simulink model "Comparision"  (R2018b)
settings: Solver=VariableStepAuto  StartTime=0.0  StopTime=40  RelTol=1e-3
values from neighbouring files (symbols this model uses):
  N = zeros(3, 7)    [InverseDynamic.m]
  s = (InverseDynamic(jointVelocity,joint ,a) - C)    [ForwardDynamicSolver.m]
undefined symbols (not defined in the file or in its folder): X, Y, Z
libraries: sm_lib x120, nesl_utility x72, simulink x1
(part 1 of 3)
settings Model: Creator=olavoie  LastModifiedBy=olavoie

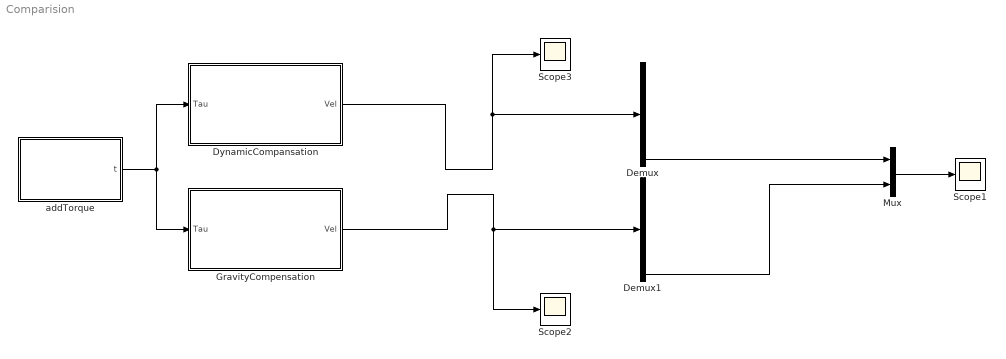
== system Comparision ==
  Demux : Demux  Outputs=7
  Demux1 : Demux  Outputs=7
  DynamicCompansation : Subsystem  TreatAsAtomicUnit=on
  GravityCompensation : Subsystem  TreatAsAtomicUnit=on
  Mux : Mux  Inputs=2
  Scope1 : Scope
  Scope2 : Scope
  Scope3 : Scope
  addTorque : Subsystem  TreatAsAtomicUnit=on
  wires:
  GravityCompensation/1(Vel) -> Demux1/1, Scope2/1
  DynamicCompansation/1(Vel) -> Demux/1, Scope3/1
  addTorque/1(t) -> DynamicCompansation/1(Tau), GravityCompensation/1(Tau)
  Demux1/7 -> Mux/2
  Demux/7 -> Mux/1
  Mux/1 -> Scope1/1

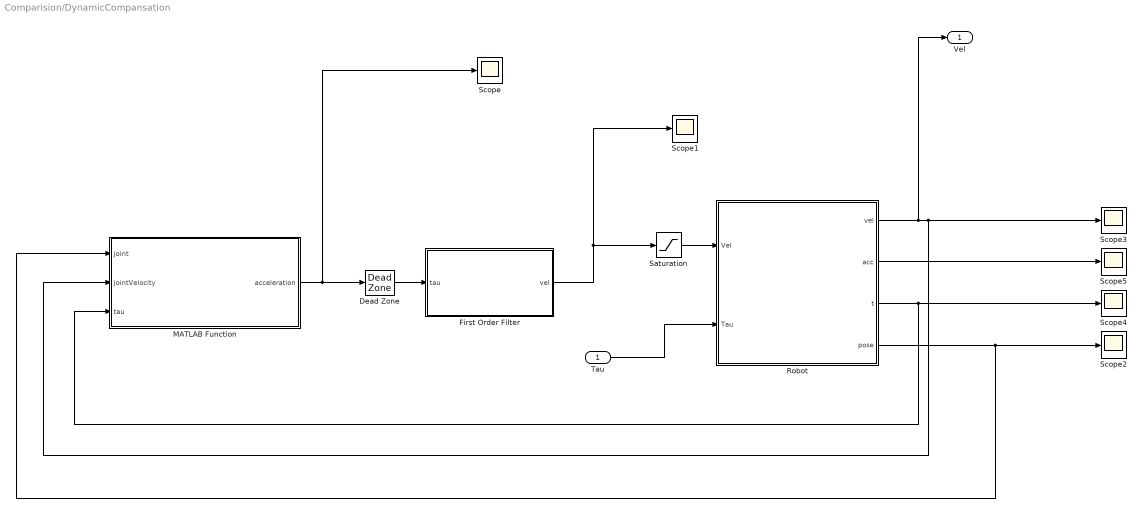
== system Comparision/DynamicCompansation ==
  Tau : Inport
  Dead Zone : DeadZone  LowerValue=-10  UpperValue=10  SaturateOnIntegerOverflow=on
  First Order Filter : Subsystem  TreatAsAtomicUnit=on
  MATLAB Function : MATLAB Function  TreatAsAtomicUnit=on
  Robot : Subsystem  TreatAsAtomicUnit=on
  Saturation : Saturate  UpperLimit=57.3  LowerLimit=-57.3
  Scope{,1..5} (6 alike) : Scope
  Vel : Outport
  wires:
  Robot/3(t) -> MATLAB Function/3(tau), Scope4/1
  Robot/4(pose) -> MATLAB Function/1(joint), Scope2/1
  MATLAB Function/1(acceleration) -> Scope/1, Dead Zone/1
  First Order Filter/1(vel) -> Saturation/1, Scope1/1
  Robot/2(acc) -> Scope5/1
  Robot/1(vel) -> Vel/1, MATLAB Function/2(jointVelocity), Scope3/1
  Dead Zone/1 -> First Order Filter/1(tau)
  Tau/1 -> Robot/2(Tau)
  Saturation/1 -> Robot/1(Vel)

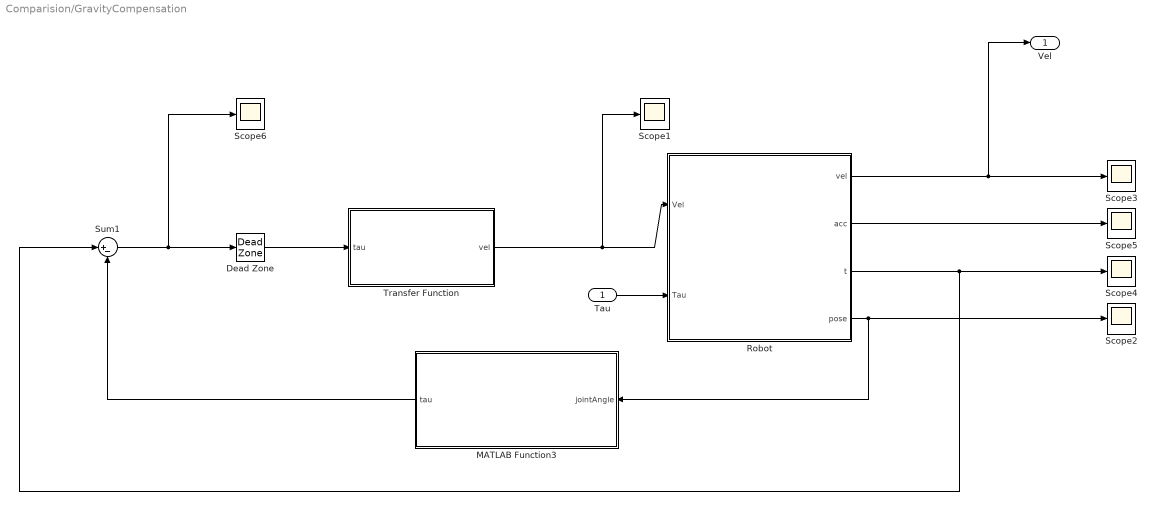
== system Comparision/GravityCompensation ==
  Tau : Inport
  Dead Zone : DeadZone  LowerValue=-10  UpperValue=10  SaturateOnIntegerOverflow=on
  MATLAB Function3 : MATLAB Function  TreatAsAtomicUnit=on
  Robot : Subsystem  TreatAsAtomicUnit=on
  Scope{1..6} (6 alike) : Scope
  Sum1 : Sum  Inputs=|+-
  Transfer Function : Subsystem  TreatAsAtomicUnit=on
  Vel : Outport
  wires:
  Robot/4(pose) -> Scope2/1, MATLAB Function3/1(jointAngle)
  Robot/2(acc) -> Scope5/1
  Robot/3(t) -> Scope4/1, Sum1/1
  Transfer Function/1(vel) -> Scope1/1, Robot/1(Vel)
  MATLAB Function3/1(tau) -> Sum1/2
  Dead Zone/1 -> Transfer Function/1(tau)
  Sum1/1 -> Scope6/1, Dead Zone/1
  Robot/1(vel) -> Vel/1, Scope3/1
  Tau/1 -> Robot/2(Tau)

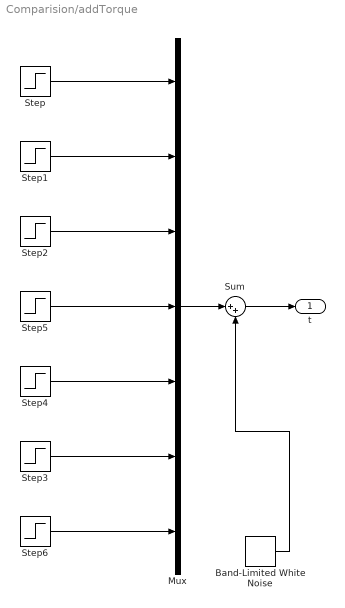
== system Comparision/addTorque ==
  Band-Limited White Noise : simulink/Sources/Band-Limited White Noise  Cov=[0.5]  Ts=0.001  seed=[23341]
  Mux : Mux  Inputs=7
  Step : Step  Time=0  After=100  SampleTime=0
  Step{1..6} (6 alike) : Step  Time=0  After=0  SampleTime=0
  Sum : Sum  Inputs=|++
  t : Outport
  wires:
  Step/1 -> Mux/1
  Step6/1 -> Mux/7
  Step3/1 -> Mux/6
  Step4/1 -> Mux/5
  Step5/1 -> Mux/4
  Step2/1 -> Mux/3
  Step1/1 -> Mux/2
  Mux/1 -> Sum/1
  Sum/1 -> t/1
  Band-Limited White Noise/1 -> Sum/2

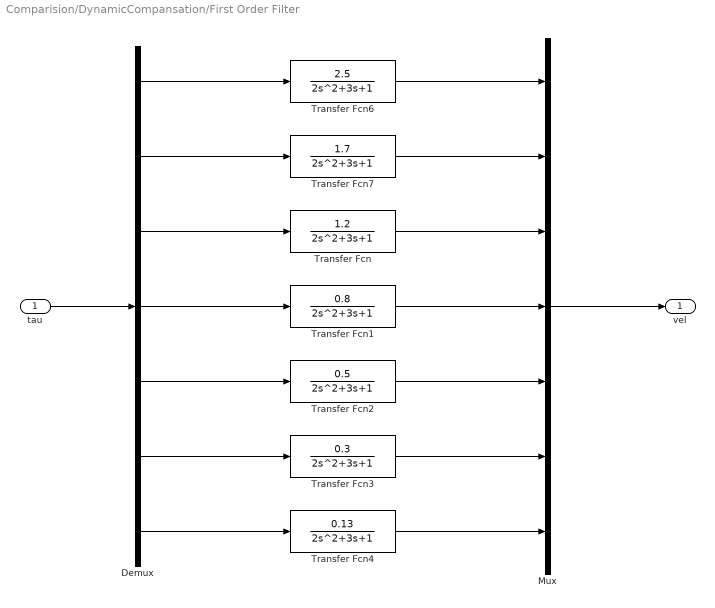
== system Comparision/DynamicCompansation/First Order Filter ==
  tau : Inport
  Demux : Demux  Outputs=7
  Mux : Mux  Inputs=7
  Transfer Fcn : TransferFcn  Numerator=[1.2]  Denominator=[2 3 1]
  Transfer Fcn1 : TransferFcn  Numerator=[0.8]  Denominator=[2 3 1]
  Transfer Fcn2 : TransferFcn  Numerator=[0.5]  Denominator=[2 3 1]
  Transfer Fcn3 : TransferFcn  Numerator=[0.3]  Denominator=[2 3 1]
  Transfer Fcn4 : TransferFcn  Numerator=[0.13]  Denominator=[2 3 1]
  Transfer Fcn6 : TransferFcn  Numerator=[2.5]  Denominator=[2 3 1]
  Transfer Fcn7 : TransferFcn  Numerator=[1.7]  Denominator=[2 3 1]
  vel : Outport
  wires:
  Transfer Fcn2/1 -> Mux/5
  Demux/7 -> Transfer Fcn4/1
  Transfer Fcn1/1 -> Mux/4
  Transfer Fcn4/1 -> Mux/7
  Transfer Fcn/1 -> Mux/3
  Demux/3 -> Transfer Fcn/1
  Demux/5 -> Transfer Fcn2/1
  Transfer Fcn7/1 -> Mux/2
  Transfer Fcn3/1 -> Mux/6
  Mux/1 -> vel/1
  Demux/4 -> Transfer Fcn1/1
  tau/1 -> Demux/1
  Demux/6 -> Transfer Fcn3/1
  Transfer Fcn6/1 -> Mux/1
  Demux/2 -> Transfer Fcn7/1
  Demux/1 -> Transfer Fcn6/1

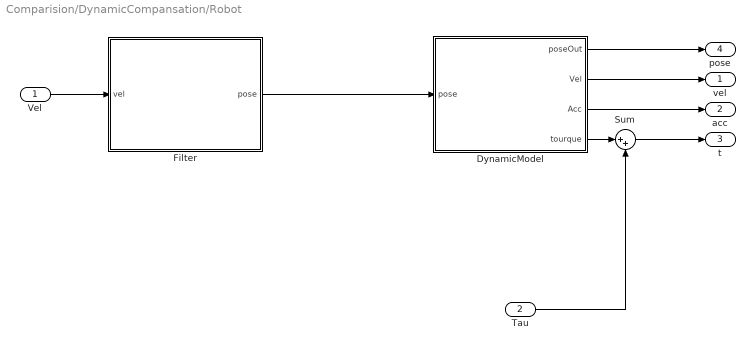
== system Comparision/DynamicCompansation/Robot ==
  Vel : Inport
  Tau : Inport  Port=2
  DynamicModel : Subsystem  TreatAsAtomicUnit=on
  Filter : Subsystem  TreatAsAtomicUnit=on
  Sum : Sum  Inputs=|++
  vel : Outport
  acc : Outport  Port=2
  t : Outport  Port=3
  pose : Outport  Port=4
  wires:
  Vel/1 -> Filter/1(vel)
  Filter/1(pose) -> DynamicModel/1(pose)
  DynamicModel/1(poseOut) -> pose/1
  DynamicModel/2(Vel) -> vel/1
  DynamicModel/3(Acc) -> acc/1
  DynamicModel/4(tourque) -> Sum/1
  Sum/1 -> t/1
  Tau/1 -> Sum/2

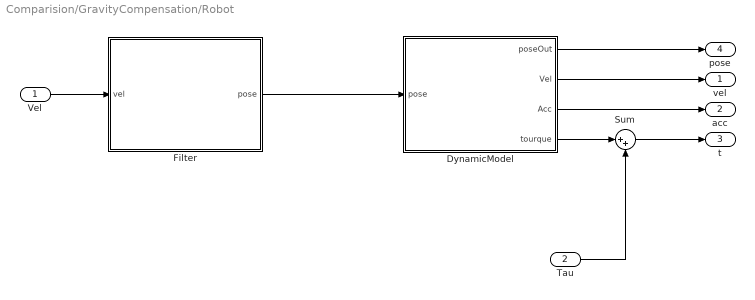
== system Comparision/GravityCompensation/Robot ==
  Vel : Inport
  Tau : Inport  Port=2
  DynamicModel : Subsystem  TreatAsAtomicUnit=on
  Filter : Subsystem  TreatAsAtomicUnit=on
  Sum : Sum  Inputs=|++
  vel : Outport
  acc : Outport  Port=2
  t : Outport  Port=3
  pose : Outport  Port=4
  wires:
  Vel/1 -> Filter/1(vel)
  Filter/1(pose) -> DynamicModel/1(pose)
  DynamicModel/1(poseOut) -> pose/1
  DynamicModel/2(Vel) -> vel/1
  DynamicModel/3(Acc) -> acc/1
  DynamicModel/4(tourque) -> Sum/1
  Sum/1 -> t/1
  Tau/1 -> Sum/2

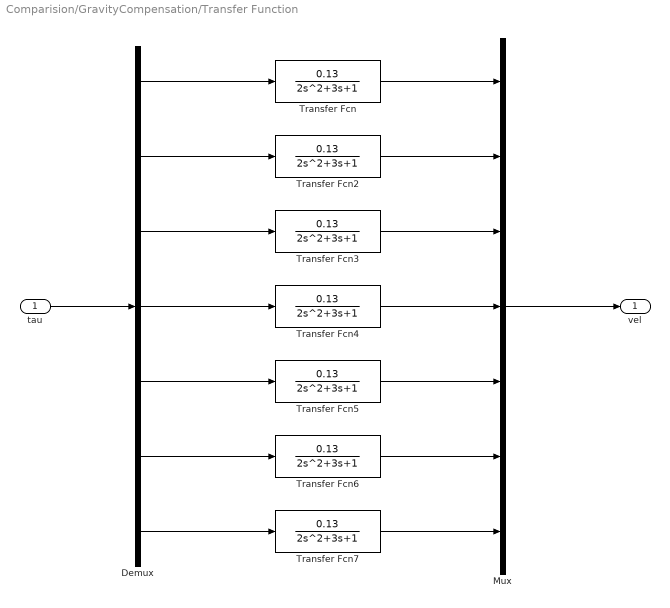
== system Comparision/GravityCompensation/Transfer Function ==
  tau : Inport
  Demux : Demux  Outputs=7
  Mux : Mux  Inputs=7
  Transfer Fcn{,2..7} (7 alike) : TransferFcn  Numerator=[0.13]  Denominator=[2 3 1]
  vel : Outport
  wires:
  Demux/1 -> Transfer Fcn/1
  Demux/2 -> Transfer Fcn2/1
  Demux/3 -> Transfer Fcn3/1
  Demux/4 -> Transfer Fcn4/1
  Demux/5 -> Transfer Fcn5/1
  Demux/6 -> Transfer Fcn6/1
  Demux/7 -> Transfer Fcn7/1
  Transfer Fcn/1 -> Mux/1
  Transfer Fcn2/1 -> Mux/2
  Transfer Fcn3/1 -> Mux/3
  Transfer Fcn4/1 -> Mux/4
  Transfer Fcn5/1 -> Mux/5
  Transfer Fcn6/1 -> Mux/6
  Transfer Fcn7/1 -> Mux/7
  tau/1 -> Demux/1
  Mux/1 -> vel/1

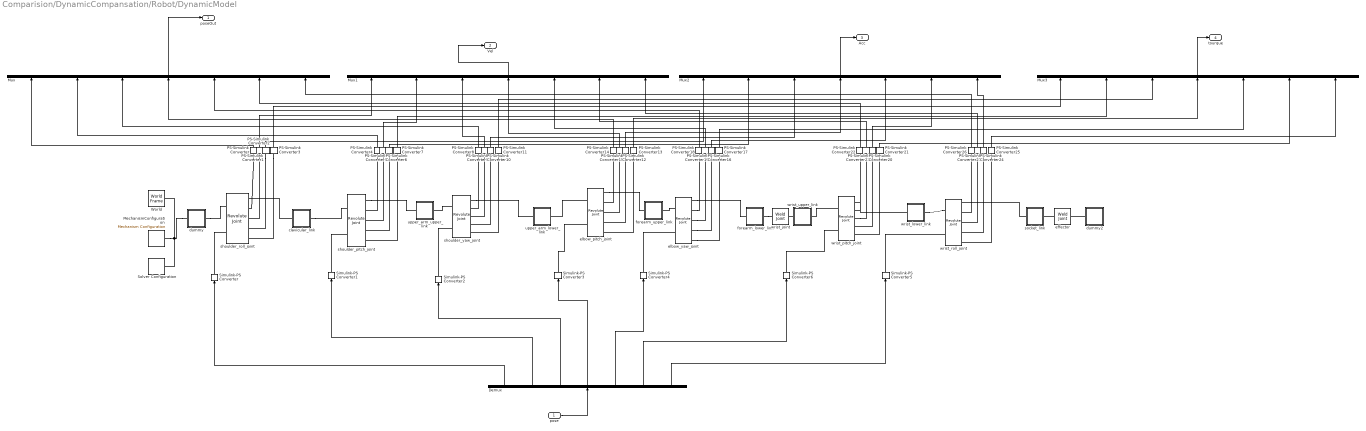
== system Comparision/DynamicCompansation/Robot/DynamicModel ==
  pose : Inport
  Demux : Demux  Outputs=7
  MechanismConfiguration : sm_lib/Utilities/Mechanism Configuration  UniformGravity=Constant  GravityVector=[0 0 -9.81]  GravityUnits=m/s^2  LinearizationDelta=0.001
  Mux{,1..3} (4 alike) : Mux  Inputs=7
  PS-Simulink Converter{,1..27} (28 alike) : nesl_utility/PS-Simulink Converter  PhysicalDomain=network_engine_domain  SubClassName=ps_output  LeftPortType=input  RightPortType=output  PseudoPeriodic=off  Frequencies=[]  Unit=1  AffineConversion=off
  Simulink-PS Converter{,1..6} (7 alike) : nesl_utility/Simulink-PS Converter  PhysicalDomain=network_engine_domain  SubClassName=ps_input  LeftPortType=input  RightPortType=output  PseudoPeriodic=off  Frequencies=[]  NoiseDistribution=none  NoiseParameters=[]  Unit=rad  AffineConversion=off  FilteringAndDerivatives=filter  SimscapeFilterOrder=2  InputFilterTimeConstant=0.001  UdotUserProvided=0
  Solver Configuration : nesl_utility/Solver Configuration  PhysicalDomain=network_engine_domain  SubClassName=solver  LeftPortType=input  RightPortType=generic  Tones=[]  Harmonics=[]  SimulateNoise=off  Profile=off  UseLocalSampling=off  EnableSwitchedLinearOptims=on  FrequencyDomain=off  UseCCode=off  RelTol=0.001  AbsTol=1e-06  MinStep=1e-09  ToWorkspace=off  RevertToSquareIcSolve=off  NumHomotopyIterations=100  PhasorMode=off  PhasorModeNumHarmonics=1  DoDC=off  ResidualTolerance=1e-09  UseLocalSolver=off  LocalSolverChoice=NE_BACKWARD_EULER_ADVANCER  LocalSolverSampleTime=0.001  DoFixedCost=off  MaxNonlinIter=3  MaxModeIter=2  LinearAlgebra=auto  EquationFormulation=NE_TIME_EF  DelaysMemoryBudget=1024  AutomaticFiltering=on  FilteringTimeConstant=0.001  PartitionStorageMethod=AS_NEEDED  PartitionMemoryBudget=1024
  World : sm_lib/Frames and Transforms/World Frame
  clavicular_link : Subsystem
  dummy : Subsystem
  dummy2 : Subsystem
  effector : sm_lib/Joints/Weld Joint  SenseConstraintForce=off  SenseConstraintForceX=off  SenseConstraintForceY=off  SenseConstraintForceZ=off  SenseConstraintTorque=off  SenseConstraintTorqueX=off  SenseConstraintTorqueY=off  SenseConstraintTorqueZ=off  SenseTotalForce=off  SenseTotalForceX=off  SenseTotalForceY=off  SenseTotalForceZ=off  SenseTotalTorque=off  SenseTotalTorqueX=off  SenseTotalTorqueY=off  SenseTotalTorqueZ=off  CompositeWrenchDir=FollowerOnBase  CompositeWrenchFrame=BaseFrame
  elbow_pitch_joint : sm_lib/Joints/Revolute Joint  SenseConstraintForce=off  SenseConstraintForceX=off  SenseConstraintForceY=off  SenseConstraintForceZ=off  SenseConstraintTorque=off  SenseConstraintTorqueX=off  SenseConstraintTorqueY=off  SenseConstraintTorqueZ=off  SenseTotalForce=off  SenseTotalForceX=off  SenseTotalForceY=off  SenseTotalForceZ=off  SenseTotalTorque=off  SenseTotalTorqueX=off  SenseTotalTorqueY=off  SenseTotalTorqueZ=off  CompositeWrenchDir=FollowerOnBase  CompositeWrenchFrame=BaseFrame  EquilibriumPosition=0  EquilibriumPositionUnits=deg  SpringStiffness=0  SpringStiffnessUnits=N*m/deg  DampingCoefficient=0.1  DampingCoefficientUnits=m^2*kg/s/rad  TorqueActuationMode=ComputedTorque  MotionActuationMode=InputMotion  SensePosition=on  SenseVelocity=on  SenseAcceleration=on  SenseTorqueForce=on  PositionTargetSpecify=off  PositionTargetPriority=High  PositionTargetValue=0  PositionTargetValueUnits=deg  VelocityTargetSpecify=off  VelocityTargetPriority=High  VelocityTargetValue=0  VelocityTargetValueUnits=deg/s
  elbow_yaw_joint : sm_lib/Joints/Revolute Joint  SenseConstraintForce=off  SenseConstraintForceX=off  SenseConstraintForceY=off  SenseConstraintForceZ=off  SenseConstraintTorque=off  SenseConstraintTorqueX=off  SenseConstraintTorqueY=off  SenseConstraintTorqueZ=off  SenseTotalForce=off  SenseTotalForceX=off  SenseTotalForceY=off  SenseTotalForceZ=off  SenseTotalTorque=off  SenseTotalTorqueX=off  SenseTotalTorqueY=off  SenseTotalTorqueZ=off  CompositeWrenchDir=FollowerOnBase  CompositeWrenchFrame=BaseFrame  EquilibriumPosition=0  EquilibriumPositionUnits=deg  SpringStiffness=0  SpringStiffnessUnits=N*m/deg  DampingCoefficient=0.1  DampingCoefficientUnits=m^2*kg/s/rad  TorqueActuationMode=ComputedTorque  MotionActuationMode=InputMotion  SensePosition=on  SenseVelocity=on  SenseAcceleration=on  SenseTorqueForce=on  PositionTargetSpecify=off  PositionTargetPriority=High  PositionTargetValue=0  PositionTargetValueUnits=deg  VelocityTargetSpecify=off  VelocityTargetPriority=High  VelocityTargetValue=0  VelocityTargetValueUnits=deg/s
  forearm_lower_link : Subsystem
  forearm_upper_link : Subsystem
  shoulder_pitch_joint : sm_lib/Joints/Revolute Joint  SenseConstraintForce=off  SenseConstraintForceX=off  SenseConstraintForceY=off  SenseConstraintForceZ=off  SenseConstraintTorque=off  SenseConstraintTorqueX=off  SenseConstraintTorqueY=off  SenseConstraintTorqueZ=off  SenseTotalForce=off  SenseTotalForceX=off  SenseTotalForceY=off  SenseTotalForceZ=off  SenseTotalTorque=off  SenseTotalTorqueX=off  SenseTotalTorqueY=off  SenseTotalTorqueZ=off  CompositeWrenchDir=FollowerOnBase  CompositeWrenchFrame=BaseFrame  EquilibriumPosition=0  EquilibriumPositionUnits=deg  SpringStiffness=0  SpringStiffnessUnits=N*m/deg  DampingCoefficient=0.1  DampingCoefficientUnits=m^2*kg/s/rad  TorqueActuationMode=ComputedTorque  MotionActuationMode=InputMotion  SensePosition=on  SenseVelocity=on  SenseAcceleration=on  SenseTorqueForce=on  PositionTargetSpecify=off  PositionTargetPriority=High  PositionTargetValue=0  PositionTargetValueUnits=deg  VelocityTargetSpecify=off  VelocityTargetPriority=High  VelocityTargetValue=0  VelocityTargetValueUnits=deg/s
  shoulder_roll_joint : sm_lib/Joints/Revolute Joint  SenseConstraintForce=off  SenseConstraintForceX=off  SenseConstraintForceY=off  SenseConstraintForceZ=off  SenseConstraintTorque=off  SenseConstraintTorqueX=off  SenseConstraintTorqueY=off  SenseConstraintTorqueZ=off  SenseTotalForce=off  SenseTotalForceX=off  SenseTotalForceY=off  SenseTotalForceZ=off  SenseTotalTorque=off  SenseTotalTorqueX=off  SenseTotalTorqueY=off  SenseTotalTorqueZ=off  CompositeWrenchDir=FollowerOnBase  CompositeWrenchFrame=FollowerFrame  EquilibriumPosition=0  EquilibriumPositionUnits=deg  SpringStiffness=0  SpringStiffnessUnits=N*m/deg  DampingCoefficient=0.1  DampingCoefficientUnits=m^2*kg/s/rad  TorqueActuationMode=ComputedTorque  MotionActuationMode=InputMotion  SensePosition=on  SenseVelocity=on  SenseAcceleration=on  SenseTorqueForce=on  PositionTargetSpecify=on  PositionTargetPriority=High  PositionTargetValue=0  PositionTargetValueUnits=deg  VelocityTargetSpecify=on  VelocityTargetPriority=High  VelocityTargetValue=0  VelocityTargetValueUnits=deg/s
  shoulder_yaw_joint : sm_lib/Joints/Revolute Joint  SenseConstraintForce=off  SenseConstraintForceX=off  SenseConstraintForceY=off  SenseConstraintForceZ=off  SenseConstraintTorque=off  SenseConstraintTorqueX=off  SenseConstraintTorqueY=off  SenseConstraintTorqueZ=off  SenseTotalForce=off  SenseTotalForceX=off  SenseTotalForceY=off  SenseTotalForceZ=off  SenseTotalTorque=off  SenseTotalTorqueX=off  SenseTotalTorqueY=off  SenseTotalTorqueZ=off  CompositeWrenchDir=FollowerOnBase  CompositeWrenchFrame=FollowerFrame  EquilibriumPosition=0  EquilibriumPositionUnits=deg  SpringStiffness=0  SpringStiffnessUnits=N*m/deg  DampingCoefficient=0.1  DampingCoefficientUnits=m^2*kg/s/rad  TorqueActuationMode=ComputedTorque  MotionActuationMode=InputMotion  SensePosition=on  SenseVelocity=on  SenseAcceleration=on  SenseTorqueForce=on  PositionTargetSpecify=off  PositionTargetPriority=High  PositionTargetValue=0  PositionTargetValueUnits=deg  VelocityTargetSpecify=off  VelocityTargetPriority=High  VelocityTargetValue=0  VelocityTargetValueUnits=deg/s
  socket_link : Subsystem
  upper_arm_lower_link : Subsystem
  upper_arm_upper_link : Subsystem
  wrist_joint : sm_lib/Joints/Weld Joint  SenseConstraintForce=off  SenseConstraintForceX=off  SenseConstraintForceY=off  SenseConstraintForceZ=off  SenseConstraintTorque=off  SenseConstraintTorqueX=off  SenseConstraintTorqueY=off  SenseConstraintTorqueZ=off  SenseTotalForce=off  SenseTotalForceX=off  SenseTotalForceY=off  SenseTotalForceZ=off  SenseTotalTorque=off  SenseTotalTorqueX=off  SenseTotalTorqueY=off  SenseTotalTorqueZ=off  CompositeWrenchDir=FollowerOnBase  CompositeWrenchFrame=BaseFrame
  wrist_lower_link : Subsystem
  wrist_pitch_joint : sm_lib/Joints/Revolute Joint  SenseConstraintForce=off  SenseConstraintForceX=off  SenseConstraintForceY=off  SenseConstraintForceZ=off  SenseConstraintTorque=off  SenseConstraintTorqueX=off  SenseConstraintTorqueY=off  SenseConstraintTorqueZ=off  SenseTotalForce=off  SenseTotalForceX=off  SenseTotalForceY=off  SenseTotalForceZ=off  SenseTotalTorque=off  SenseTotalTorqueX=off  SenseTotalTorqueY=off  SenseTotalTorqueZ=off  CompositeWrenchDir=FollowerOnBase  CompositeWrenchFrame=BaseFrame  EquilibriumPosition=0  EquilibriumPositionUnits=deg  SpringStiffness=0  SpringStiffnessUnits=N*m/deg  DampingCoefficient=0.1  DampingCoefficientUnits=m^2*kg/s/rad  TorqueActuationMode=ComputedTorque  MotionActuationMode=InputMotion  SensePosition=on  SenseVelocity=on  SenseAcceleration=on  SenseTorqueForce=on  PositionTargetSpecify=off  PositionTargetPriority=High  PositionTargetValue=0  PositionTargetValueUnits=deg  VelocityTargetSpecify=off  VelocityTargetPriority=High  VelocityTargetValue=0  VelocityTargetValueUnits=deg/s
  wrist_roll_joint : sm_lib/Joints/Revolute Joint  SenseConstraintForce=off  SenseConstraintForceX=off  SenseConstraintForceY=off  SenseConstraintForceZ=off  SenseConstraintTorque=off  SenseConstraintTorqueX=off  SenseConstraintTorqueY=off  SenseConstraintTorqueZ=off  SenseTotalForce=off  SenseTotalForceX=off  SenseTotalForceY=off  SenseTotalForceZ=off  SenseTotalTorque=off  SenseTotalTorqueX=off  SenseTotalTorqueY=off  SenseTotalTorqueZ=off  CompositeWrenchDir=FollowerOnBase  CompositeWrenchFrame=BaseFrame  EquilibriumPosition=0  EquilibriumPositionUnits=deg  SpringStiffness=0  SpringStiffnessUnits=N*m/deg  DampingCoefficient=0.1  DampingCoefficientUnits=m^2*kg/s/rad  TorqueActuationMode=ComputedTorque  MotionActuationMode=InputMotion  SensePosition=on  SenseVelocity=on  SenseAcceleration=on  SenseTorqueForce=on  PositionTargetSpecify=off  PositionTargetPriority=High  PositionTargetValue=0  PositionTargetValueUnits=deg  VelocityTargetSpecify=off  VelocityTargetPriority=High  VelocityTargetValue=0  VelocityTargetValueUnits=deg/s
  wrist_upper_link : Subsystem
  poseOut : Outport
  Vel : Outport  Port=2
  Acc : Outport  Port=3
  tourque : Outport  Port=4
  wires:
  PS-Simulink Converter23/1 -> Mux1/6
  PS-Simulink Converter25/1 -> Mux3/7
  PS-Simulink Converter12/1 -> Mux2/4
  PS-Simulink Converter16/1 -> Mux2/5
  Mux1/1 -> Vel/1
  PS-Simulink Converter19/1 -> Mux1/5
  PS-Simulink Converter27/1 -> Mux1/7
  Demux/7 -> Simulink-PS Converter5/1
  PS-Simulink Converter/1 -> Mux/1
  PS-Simulink Converter20/1 -> Mux2/6
  Mux3/1 -> tourque/1
  Demux/1 -> Simulink-PS Converter/1
  PS-Simulink Converter22/1 -> Mux/6
  Mux2/1 -> Acc/1
  PS-Simulink Converter7/1 -> Mux3/2
  PS-Simulink Converter26/1 -> Mux/7
  PS-Simulink Converter10/1 -> Mux2/3
  Demux/6 -> Simulink-PS Converter6/1
  PS-Simulink Converter18/1 -> Mux/5
  PS-Simulink Converter24/1 -> Mux2/7
  PS-Simulink Converter14/1 -> Mux/4
  PS-Simulink Converter5/1 -> Mux1/2
  PS-Simulink Converter17/1 -> Mux3/5
  PS-Simulink Converter21/1 -> Mux3/6
  Demux/5 -> Simulink-PS Converter4/1
  PS-Simulink Converter2/1 -> Mux2/1
  PS-Simulink Converter8/1 -> Mux/3
  PS-Simulink Converter13/1 -> Mux3/4
  PS-Simulink Converter11/1 -> Mux3/3
  Mux/1 -> poseOut/1
  PS-Simulink Converter9/1 -> Mux1/3
  PS-Simulink Converter15/1 -> Mux1/4
  PS-Simulink Converter3/1 -> Mux3/1
  PS-Simulink Converter1/1 -> Mux1/1
  PS-Simulink Converter6/1 -> Mux2/2
  Demux/2 -> Simulink-PS Converter1/1
  PS-Simulink Converter4/1 -> Mux/2
  Demux/3 -> Simulink-PS Converter2/1
  pose/1 -> Demux/1
  Demux/4 -> Simulink-PS Converter3/1
  connections:
  dummy/LConn1 -- MechanismConfiguration/RConn1 -- Solver Configuration/RConn1 -- World/RConn1
  elbow_yaw_joint/RConn1 -- forearm_lower_link/LConn1
  PS-Simulink Converter3/LConn1 -- shoulder_roll_joint/RConn5
  elbow_yaw_joint/RConn5 -- PS-Simulink Converter17/LConn1
  PS-Simulink Converter6/LConn1 -- shoulder_pitch_joint/RConn4
  wrist_lower_link/LConn1 -- wrist_pitch_joint/RConn1
  PS-Simulink Converter14/LConn1 -- elbow_pitch_joint/RConn2
  PS-Simulink Converter5/LConn1 -- shoulder_pitch_joint/RConn3
  shoulder_yaw_joint/LConn2 -- Simulink-PS Converter2/RConn1
  clavicular_link/LConn1 -- shoulder_roll_joint/RConn1
  PS-Simulink Converter12/LConn1 -- elbow_pitch_joint/RConn4
  wrist_pitch_joint/RConn2 -- PS-Simulink Converter22/LConn1
  PS-Simulink Converter24/LConn1 -- wrist_roll_joint/RConn4
  Simulink-PS Converter6/RConn1 -- wrist_pitch_joint/LConn2
  PS-Simulink Converter4/LConn1 -- shoulder_pitch_joint/RConn2
  PS-Simulink Converter21/LConn1 -- wrist_pitch_joint/RConn5
  PS-Simulink Converter13/LConn1 -- elbow_pitch_joint/RConn5
  socket_link/LConn1 -- wrist_roll_joint/RConn1
  PS-Simulink Converter/LConn1 -- shoulder_roll_joint/RConn2
  PS-Simulink Converter2/LConn1 -- shoulder_roll_joint/RConn4
  elbow_yaw_joint/RConn2 -- PS-Simulink Converter18/LConn1
  PS-Simulink Converter1/LConn1 -- shoulder_roll_joint/RConn3
  PS-Simulink Converter25/LConn1 -- wrist_roll_joint/RConn5
  shoulder_pitch_joint/RConn1 -- upper_arm_upper_link/LConn1
  PS-Simulink Converter10/LConn1 -- shoulder_yaw_joint/RConn4
  PS-Simulink Converter7/LConn1 -- shoulder_pitch_joint/RConn5
  elbow_pitch_joint/LConn2 -- Simulink-PS Converter3/RConn1
  PS-Simulink Converter27/LConn1 -- wrist_roll_joint/RConn3
  dummy2/LConn1 -- effector/RConn1
  elbow_yaw_joint/RConn3 -- PS-Simulink Converter19/LConn1
  shoulder_yaw_joint/RConn1 -- upper_arm_lower_link/LConn1
  PS-Simulink Converter11/LConn1 -- shoulder_yaw_joint/RConn5
  wrist_lower_link/RConn1 -- wrist_roll_joint/LConn1
  PS-Simulink Converter26/LConn1 -- wrist_roll_joint/RConn2
  shoulder_yaw_joint/LConn1 -- upper_arm_upper_link/RConn1
  wrist_joint/RConn1 -- wrist_upper_link/LConn1
  PS-Simulink Converter20/LConn1 -- wrist_pitch_joint/RConn4
  elbow_yaw_joint/LConn2 -- Simulink-PS Converter4/RConn1
  forearm_lower_link/RConn1 -- wrist_joint/LConn1
  effector/LConn1 -- socket_link/RConn1
  Simulink-PS Converter1/RConn1 -- shoulder_pitch_joint/LConn2
  elbow_pitch_joint/RConn1 -- forearm_upper_link/LConn1
  elbow_pitch_joint/LConn1 -- upper_arm_lower_link/RConn1
  dummy/RConn1 -- shoulder_roll_joint/LConn1
  PS-Simulink Converter15/LConn1 -- elbow_pitch_joint/RConn3
  wrist_pitch_joint/RConn3 -- PS-Simulink Converter23/LConn1
  elbow_yaw_joint/RConn4 -- PS-Simulink Converter16/LConn1
  clavicular_link/RConn1 -- shoulder_pitch_joint/LConn1
  Simulink-PS Converter5/RConn1 -- wrist_roll_joint/LConn2
  wrist_pitch_joint/LConn1 -- wrist_upper_link/RConn1
  PS-Simulink Converter8/LConn1 -- shoulder_yaw_joint/RConn2
  PS-Simulink Converter9/LConn1 -- shoulder_yaw_joint/RConn3
  elbow_yaw_joint/LConn1 -- forearm_upper_link/RConn1
  Simulink-PS Converter/RConn1 -- shoulder_roll_joint/LConn2

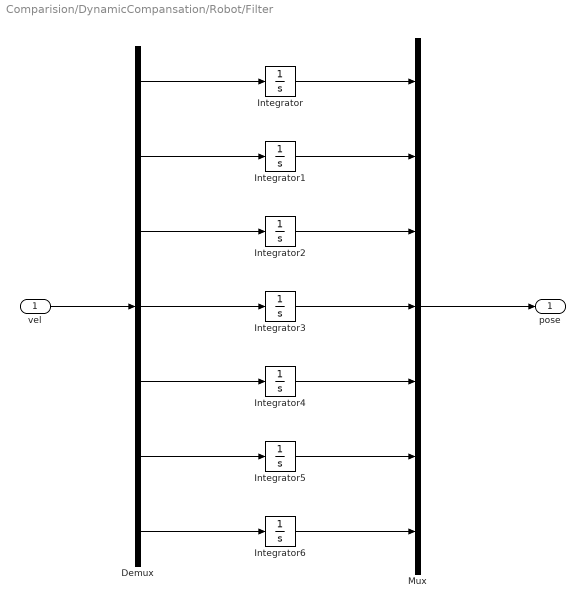
== system Comparision/DynamicCompansation/Robot/Filter ==
  vel : Inport
  Demux : Demux  Outputs=7
  Integrator{,1..6} (7 alike) : Integrator
  Mux : Mux  Inputs=7
  pose : Outport
  wires:
  Mux/1 -> pose/1
  Demux/1 -> Integrator/1
  Integrator/1 -> Mux/1
  Demux/7 -> Integrator6/1
  Integrator6/1 -> Mux/7
  Demux/6 -> Integrator5/1
  Integrator5/1 -> Mux/6
  Demux/5 -> Integrator4/1
  Integrator4/1 -> Mux/5
  Demux/4 -> Integrator3/1
  Integrator3/1 -> Mux/4
  Demux/3 -> Integrator2/1
  Integrator2/1 -> Mux/3
  Demux/2 -> Integrator1/1
  Integrator1/1 -> Mux/2
  vel/1 -> Demux/1

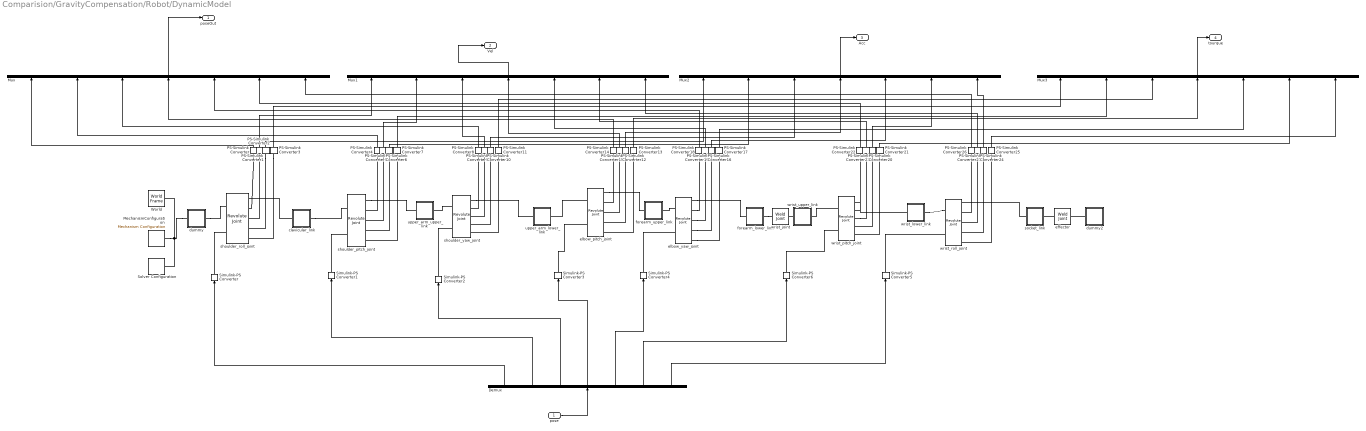
== system Comparision/GravityCompensation/Robot/DynamicModel ==
  pose : Inport
  Demux : Demux  Outputs=7
  MechanismConfiguration : sm_lib/Utilities/Mechanism Configuration  UniformGravity=Constant  GravityVector=[0 0 9.81]  GravityUnits=m/s^2  LinearizationDelta=0.001
  Mux{,1..3} (4 alike) : Mux  Inputs=7
  PS-Simulink Converter{,1..27} (28 alike) : nesl_utility/PS-Simulink Converter  PhysicalDomain=network_engine_domain  SubClassName=ps_output  LeftPortType=input  RightPortType=output  PseudoPeriodic=off  Frequencies=[]  Unit=1  AffineConversion=off
  Simulink-PS Converter{,1..6} (7 alike) : nesl_utility/Simulink-PS Converter  PhysicalDomain=network_engine_domain  SubClassName=ps_input  LeftPortType=input  RightPortType=output  PseudoPeriodic=off  Frequencies=[]  NoiseDistribution=none  NoiseParameters=[]  Unit=rad  AffineConversion=off  FilteringAndDerivatives=filter  SimscapeFilterOrder=2  InputFilterTimeConstant=0.001  UdotUserProvided=0
  Solver Configuration : nesl_utility/Solver Configuration  PhysicalDomain=network_engine_domain  SubClassName=solver  LeftPortType=input  RightPortType=generic  Tones=[]  Harmonics=[]  SimulateNoise=off  Profile=off  UseLocalSampling=off  EnableSwitchedLinearOptims=on  FrequencyDomain=off  UseCCode=off  RelTol=0.001  AbsTol=1e-06  MinStep=1e-09  ToWorkspace=off  RevertToSquareIcSolve=off  NumHomotopyIterations=100  PhasorMode=off  PhasorModeNumHarmonics=1  DoDC=off  ResidualTolerance=1e-09  UseLocalSolver=off  LocalSolverChoice=NE_BACKWARD_EULER_ADVANCER  LocalSolverSampleTime=0.001  DoFixedCost=off  MaxNonlinIter=3  MaxModeIter=2  LinearAlgebra=auto  EquationFormulation=NE_TIME_EF  DelaysMemoryBudget=1024  AutomaticFiltering=on  FilteringTimeConstant=0.001  PartitionStorageMethod=AS_NEEDED  PartitionMemoryBudget=1024
  World : sm_lib/Frames and Transforms/World Frame
  clavicular_link : Subsystem
  dummy : Subsystem
  dummy2 : Subsystem
  effector : sm_lib/Joints/Weld Joint  SenseConstraintForce=off  SenseConstraintForceX=off  SenseConstraintForceY=off  SenseConstraintForceZ=off  SenseConstraintTorque=off  SenseConstraintTorqueX=off  SenseConstraintTorqueY=off  SenseConstraintTorqueZ=off  SenseTotalForce=off  SenseTotalForceX=off  SenseTotalForceY=off  SenseTotalForceZ=off  SenseTotalTorque=off  SenseTotalTorqueX=off  SenseTotalTorqueY=off  SenseTotalTorqueZ=off  CompositeWrenchDir=FollowerOnBase  CompositeWrenchFrame=BaseFrame
  elbow_pitch_joint : sm_lib/Joints/Revolute Joint  SenseConstraintForce=off  SenseConstraintForceX=off  SenseConstraintForceY=off  SenseConstraintForceZ=off  SenseConstraintTorque=off  SenseConstraintTorqueX=off  SenseConstraintTorqueY=off  SenseConstraintTorqueZ=off  SenseTotalForce=off  SenseTotalForceX=off  SenseTotalForceY=off  SenseTotalForceZ=off  SenseTotalTorque=off  SenseTotalTorqueX=off  SenseTotalTorqueY=off  SenseTotalTorqueZ=off  CompositeWrenchDir=FollowerOnBase  CompositeWrenchFrame=BaseFrame  EquilibriumPosition=0  EquilibriumPositionUnits=deg  SpringStiffness=0  SpringStiffnessUnits=N*m/deg  DampingCoefficient=0.1  DampingCoefficientUnits=m^2*kg/s/rad  TorqueActuationMode=ComputedTorque  MotionActuationMode=InputMotion  SensePosition=on  SenseVelocity=on  SenseAcceleration=on  SenseTorqueForce=on  PositionTargetSpecify=off  PositionTargetPriority=High  PositionTargetValue=0  PositionTargetValueUnits=deg  VelocityTargetSpecify=off  VelocityTargetPriority=High  VelocityTargetValue=0  VelocityTargetValueUnits=deg/s
  elbow_yaw_joint : sm_lib/Joints/Revolute Joint  SenseConstraintForce=off  SenseConstraintForceX=off  SenseConstraintForceY=off  SenseConstraintForceZ=off  SenseConstraintTorque=off  SenseConstraintTorqueX=off  SenseConstraintTorqueY=off  SenseConstraintTorqueZ=off  SenseTotalForce=off  SenseTotalForceX=off  SenseTotalForceY=off  SenseTotalForceZ=off  SenseTotalTorque=off  SenseTotalTorqueX=off  SenseTotalTorqueY=off  SenseTotalTorqueZ=off  CompositeWrenchDir=FollowerOnBase  CompositeWrenchFrame=BaseFrame  EquilibriumPosition=0  EquilibriumPositionUnits=deg  SpringStiffness=0  SpringStiffnessUnits=N*m/deg  DampingCoefficient=0.1  DampingCoefficientUnits=m^2*kg/s/rad  TorqueActuationMode=ComputedTorque  MotionActuationMode=InputMotion  SensePosition=on  SenseVelocity=on  SenseAcceleration=on  SenseTorqueForce=on  PositionTargetSpecify=off  PositionTargetPriority=High  PositionTargetValue=0  PositionTargetValueUnits=deg  VelocityTargetSpecify=off  VelocityTargetPriority=High  VelocityTargetValue=0  VelocityTargetValueUnits=deg/s
  forearm_lower_link : Subsystem
  forearm_upper_link : Subsystem
  shoulder_pitch_joint : sm_lib/Joints/Revolute Joint  SenseConstraintForce=off  SenseConstraintForceX=off  SenseConstraintForceY=off  SenseConstraintForceZ=off  SenseConstraintTorque=off  SenseConstraintTorqueX=off  SenseConstraintTorqueY=off  SenseConstraintTorqueZ=off  SenseTotalForce=off  SenseTotalForceX=off  SenseTotalForceY=off  SenseTotalForceZ=off  SenseTotalTorque=off  SenseTotalTorqueX=off  SenseTotalTorqueY=off  SenseTotalTorqueZ=off  CompositeWrenchDir=FollowerOnBase  CompositeWrenchFrame=BaseFrame  EquilibriumPosition=0  EquilibriumPositionUnits=deg  SpringStiffness=0  SpringStiffnessUnits=N*m/deg  DampingCoefficient=0.1  DampingCoefficientUnits=m^2*kg/s/rad  TorqueActuationMode=ComputedTorque  MotionActuationMode=InputMotion  SensePosition=on  SenseVelocity=on  SenseAcceleration=on  SenseTorqueForce=on  PositionTargetSpecify=off  PositionTargetPriority=High  PositionTargetValue=0  PositionTargetValueUnits=deg  VelocityTargetSpecify=off  VelocityTargetPriority=High  VelocityTargetValue=0  VelocityTargetValueUnits=deg/s
  shoulder_roll_joint : sm_lib/Joints/Revolute Joint  SenseConstraintForce=off  SenseConstraintForceX=off  SenseConstraintForceY=off  SenseConstraintForceZ=off  SenseConstraintTorque=off  SenseConstraintTorqueX=off  SenseConstraintTorqueY=off  SenseConstraintTorqueZ=off  SenseTotalForce=off  SenseTotalForceX=off  SenseTotalForceY=off  SenseTotalForceZ=off  SenseTotalTorque=off  SenseTotalTorqueX=off  SenseTotalTorqueY=off  SenseTotalTorqueZ=off  CompositeWrenchDir=FollowerOnBase  CompositeWrenchFrame=FollowerFrame  EquilibriumPosition=0  EquilibriumPositionUnits=deg  SpringStiffness=0  SpringStiffnessUnits=N*m/deg  DampingCoefficient=0.1  DampingCoefficientUnits=m^2*kg/s/rad  TorqueActuationMode=ComputedTorque  MotionActuationMode=InputMotion  SensePosition=on  SenseVelocity=on  SenseAcceleration=on  SenseTorqueForce=on  PositionTargetSpecify=on  PositionTargetPriority=High  PositionTargetValue=0  PositionTargetValueUnits=deg  VelocityTargetSpecify=on  VelocityTargetPriority=High  VelocityTargetValue=0  VelocityTargetValueUnits=deg/s
  shoulder_yaw_joint : sm_lib/Joints/Revolute Joint  SenseConstraintForce=off  SenseConstraintForceX=off  SenseConstraintForceY=off  SenseConstraintForceZ=off  SenseConstraintTorque=off  SenseConstraintTorqueX=off  SenseConstraintTorqueY=off  SenseConstraintTorqueZ=off  SenseTotalForce=off  SenseTotalForceX=off  SenseTotalForceY=off  SenseTotalForceZ=off  SenseTotalTorque=off  SenseTotalTorqueX=off  SenseTotalTorqueY=off  SenseTotalTorqueZ=off  CompositeWrenchDir=FollowerOnBase  CompositeWrenchFrame=FollowerFrame  EquilibriumPosition=0  EquilibriumPositionUnits=deg  SpringStiffness=0  SpringStiffnessUnits=N*m/deg  DampingCoefficient=0.1  DampingCoefficientUnits=m^2*kg/s/rad  TorqueActuationMode=ComputedTorque  MotionActuationMode=InputMotion  SensePosition=on  SenseVelocity=on  SenseAcceleration=on  SenseTorqueForce=on  PositionTargetSpecify=off  PositionTargetPriority=High  PositionTargetValue=0  PositionTargetValueUnits=deg  VelocityTargetSpecify=off  VelocityTargetPriority=High  VelocityTargetValue=0  VelocityTargetValueUnits=deg/s
  socket_link : Subsystem
  upper_arm_lower_link : Subsystem
  upper_arm_upper_link : Subsystem
  wrist_joint : sm_lib/Joints/Weld Joint  SenseConstraintForce=off  SenseConstraintForceX=off  SenseConstraintForceY=off  SenseConstraintForceZ=off  SenseConstraintTorque=off  SenseConstraintTorqueX=off  SenseConstraintTorqueY=off  SenseConstraintTorqueZ=off  SenseTotalForce=off  SenseTotalForceX=off  SenseTotalForceY=off  SenseTotalForceZ=off  SenseTotalTorque=off  SenseTotalTorqueX=off  SenseTotalTorqueY=off  SenseTotalTorqueZ=off  CompositeWrenchDir=FollowerOnBase  CompositeWrenchFrame=BaseFrame
  wrist_lower_link : Subsystem
  wrist_pitch_joint : sm_lib/Joints/Revolute Joint  SenseConstraintForce=off  SenseConstraintForceX=off  SenseConstraintForceY=off  SenseConstraintForceZ=off  SenseConstraintTorque=off  SenseConstraintTorqueX=off  SenseConstraintTorqueY=off  SenseConstraintTorqueZ=off  SenseTotalForce=off  SenseTotalForceX=off  SenseTotalForceY=off  SenseTotalForceZ=off  SenseTotalTorque=off  SenseTotalTorqueX=off  SenseTotalTorqueY=off  SenseTotalTorqueZ=off  CompositeWrenchDir=FollowerOnBase  CompositeWrenchFrame=BaseFrame  EquilibriumPosition=0  EquilibriumPositionUnits=deg  SpringStiffness=0  SpringStiffnessUnits=N*m/deg  DampingCoefficient=0.1  DampingCoefficientUnits=m^2*kg/s/rad  TorqueActuationMode=ComputedTorque  MotionActuationMode=InputMotion  SensePosition=on  SenseVelocity=on  SenseAcceleration=on  SenseTorqueForce=on  PositionTargetSpecify=off  PositionTargetPriority=High  PositionTargetValue=0  PositionTargetValueUnits=deg  VelocityTargetSpecify=off  VelocityTargetPriority=High  VelocityTargetValue=0  VelocityTargetValueUnits=deg/s
  wrist_roll_joint : sm_lib/Joints/Revolute Joint  SenseConstraintForce=off  SenseConstraintForceX=off  SenseConstraintForceY=off  SenseConstraintForceZ=off  SenseConstraintTorque=off  SenseConstraintTorqueX=off  SenseConstraintTorqueY=off  SenseConstraintTorqueZ=off  SenseTotalForce=off  SenseTotalForceX=off  SenseTotalForceY=off  SenseTotalForceZ=off  SenseTotalTorque=off  SenseTotalTorqueX=off  SenseTotalTorqueY=off  SenseTotalTorqueZ=off  CompositeWrenchDir=FollowerOnBase  CompositeWrenchFrame=BaseFrame  EquilibriumPosition=0  EquilibriumPositionUnits=deg  SpringStiffness=0  SpringStiffnessUnits=N*m/deg  DampingCoefficient=0.1  DampingCoefficientUnits=m^2*kg/s/rad  TorqueActuationMode=ComputedTorque  MotionActuationMode=InputMotion  SensePosition=on  SenseVelocity=on  SenseAcceleration=on  SenseTorqueForce=on  PositionTargetSpecify=off  PositionTargetPriority=High  PositionTargetValue=0  PositionTargetValueUnits=deg  VelocityTargetSpecify=off  VelocityTargetPriority=High  VelocityTargetValue=0  VelocityTargetValueUnits=deg/s
  wrist_upper_link : Subsystem
  poseOut : Outport
  Vel : Outport  Port=2
  Acc : Outport  Port=3
  tourque : Outport  Port=4
  wires:
  PS-Simulink Converter23/1 -> Mux1/6
  PS-Simulink Converter25/1 -> Mux3/7
  PS-Simulink Converter12/1 -> Mux2/4
  PS-Simulink Converter16/1 -> Mux2/5
  Mux1/1 -> Vel/1
  PS-Simulink Converter19/1 -> Mux1/5
  PS-Simulink Converter27/1 -> Mux1/7
  Demux/7 -> Simulink-PS Converter5/1
  PS-Simulink Converter/1 -> Mux/1
  PS-Simulink Converter20/1 -> Mux2/6
  Mux3/1 -> tourque/1
  Demux/1 -> Simulink-PS Converter/1
  PS-Simulink Converter22/1 -> Mux/6
  Mux2/1 -> Acc/1
  PS-Simulink Converter7/1 -> Mux3/2
  PS-Simulink Converter26/1 -> Mux/7
  PS-Simulink Converter10/1 -> Mux2/3
  Demux/6 -> Simulink-PS Converter6/1
  PS-Simulink Converter18/1 -> Mux/5
  PS-Simulink Converter24/1 -> Mux2/7
  PS-Simulink Converter14/1 -> Mux/4
  PS-Simulink Converter5/1 -> Mux1/2
  PS-Simulink Converter17/1 -> Mux3/5
  PS-Simulink Converter21/1 -> Mux3/6
  Demux/5 -> Simulink-PS Converter4/1
  PS-Simulink Converter2/1 -> Mux2/1
  PS-Simulink Converter8/1 -> Mux/3
  PS-Simulink Converter13/1 -> Mux3/4
  PS-Simulink Converter11/1 -> Mux3/3
  Mux/1 -> poseOut/1
  PS-Simulink Converter9/1 -> Mux1/3
  PS-Simulink Converter15/1 -> Mux1/4
  PS-Simulink Converter3/1 -> Mux3/1
  PS-Simulink Converter1/1 -> Mux1/1
  PS-Simulink Converter6/1 -> Mux2/2
  Demux/2 -> Simulink-PS Converter1/1
  PS-Simulink Converter4/1 -> Mux/2
  Demux/3 -> Simulink-PS Converter2/1
  pose/1 -> Demux/1
  Demux/4 -> Simulink-PS Converter3/1
  connections:
  dummy/LConn1 -- MechanismConfiguration/RConn1 -- Solver Configuration/RConn1 -- World/RConn1
  elbow_yaw_joint/RConn1 -- forearm_lower_link/LConn1
  PS-Simulink Converter3/LConn1 -- shoulder_roll_joint/RConn5
  elbow_yaw_joint/RConn5 -- PS-Simulink Converter17/LConn1
  PS-Simulink Converter6/LConn1 -- shoulder_pitch_joint/RConn4
  wrist_lower_link/LConn1 -- wrist_pitch_joint/RConn1
  PS-Simulink Converter14/LConn1 -- elbow_pitch_joint/RConn2
  PS-Simulink Converter5/LConn1 -- shoulder_pitch_joint/RConn3
  shoulder_yaw_joint/LConn2 -- Simulink-PS Converter2/RConn1
  clavicular_link/LConn1 -- shoulder_roll_joint/RConn1
  PS-Simulink Converter12/LConn1 -- elbow_pitch_joint/RConn4
  wrist_pitch_joint/RConn2 -- PS-Simulink Converter22/LConn1
  PS-Simulink Converter24/LConn1 -- wrist_roll_joint/RConn4
  Simulink-PS Converter6/RConn1 -- wrist_pitch_joint/LConn2
  PS-Simulink Converter4/LConn1 -- shoulder_pitch_joint/RConn2
  PS-Simulink Converter21/LConn1 -- wrist_pitch_joint/RConn5
  PS-Simulink Converter13/LConn1 -- elbow_pitch_joint/RConn5
  socket_link/LConn1 -- wrist_roll_joint/RConn1
  PS-Simulink Converter/LConn1 -- shoulder_roll_joint/RConn2
  PS-Simulink Converter2/LConn1 -- shoulder_roll_joint/RConn4
  elbow_yaw_joint/RConn2 -- PS-Simulink Converter18/LConn1
  PS-Simulink Converter1/LConn1 -- shoulder_roll_joint/RConn3
  PS-Simulink Converter25/LConn1 -- wrist_roll_joint/RConn5
  shoulder_pitch_joint/RConn1 -- upper_arm_upper_link/LConn1
  PS-Simulink Converter10/LConn1 -- shoulder_yaw_joint/RConn4
  PS-Simulink Converter7/LConn1 -- shoulder_pitch_joint/RConn5
  elbow_pitch_joint/LConn2 -- Simulink-PS Converter3/RConn1
  PS-Simulink Converter27/LConn1 -- wrist_roll_joint/RConn3
  dummy2/LConn1 -- effector/RConn1
  elbow_yaw_joint/RConn3 -- PS-Simulink Converter19/LConn1
  shoulder_yaw_joint/RConn1 -- upper_arm_lower_link/LConn1
  PS-Simulink Converter11/LConn1 -- shoulder_yaw_joint/RConn5
  wrist_lower_link/RConn1 -- wrist_roll_joint/LConn1
  PS-Simulink Converter26/LConn1 -- wrist_roll_joint/RConn2
  shoulder_yaw_joint/LConn1 -- upper_arm_upper_link/RConn1
  wrist_joint/RConn1 -- wrist_upper_link/LConn1
  PS-Simulink Converter20/LConn1 -- wrist_pitch_joint/RConn4
  elbow_yaw_joint/LConn2 -- Simulink-PS Converter4/RConn1
  forearm_lower_link/RConn1 -- wrist_joint/LConn1
  effector/LConn1 -- socket_link/RConn1
  Simulink-PS Converter1/RConn1 -- shoulder_pitch_joint/LConn2
  elbow_pitch_joint/RConn1 -- forearm_upper_link/LConn1
  elbow_pitch_joint/LConn1 -- upper_arm_lower_link/RConn1
  dummy/RConn1 -- shoulder_roll_joint/LConn1
  PS-Simulink Converter15/LConn1 -- elbow_pitch_joint/RConn3
  wrist_pitch_joint/RConn3 -- PS-Simulink Converter23/LConn1
  elbow_yaw_joint/RConn4 -- PS-Simulink Converter16/LConn1
  clavicular_link/RConn1 -- shoulder_pitch_joint/LConn1
  Simulink-PS Converter5/RConn1 -- wrist_roll_joint/LConn2
  wrist_pitch_joint/LConn1 -- wrist_upper_link/RConn1
  PS-Simulink Converter8/LConn1 -- shoulder_yaw_joint/RConn2
  PS-Simulink Converter9/LConn1 -- shoulder_yaw_joint/RConn3
  elbow_yaw_joint/LConn1 -- forearm_upper_link/RConn1
  Simulink-PS Converter/RConn1 -- shoulder_roll_joint/LConn2

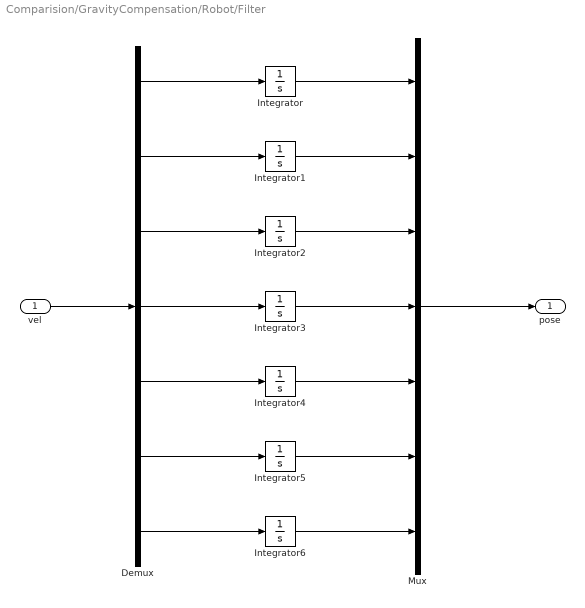
== system Comparision/GravityCompensation/Robot/Filter ==
  vel : Inport
  Demux : Demux  Outputs=7
  Integrator{,1..6} (7 alike) : Integrator
  Mux : Mux  Inputs=7
  pose : Outport
  wires:
  Mux/1 -> pose/1
  Demux/1 -> Integrator/1
  Integrator/1 -> Mux/1
  Demux/7 -> Integrator6/1
  Integrator6/1 -> Mux/7
  Demux/6 -> Integrator5/1
  Integrator5/1 -> Mux/6
  Demux/5 -> Integrator4/1
  Integrator4/1 -> Mux/5
  Demux/4 -> Integrator3/1
  Integrator3/1 -> Mux/4
  Demux/3 -> Integrator2/1
  Integrator2/1 -> Mux/3
  Demux/2 -> Integrator1/1
  Integrator1/1 -> Mux/2
  vel/1 -> Demux/1

== system Comparision/DynamicCompansation/Robot/DynamicModel/clavicular_link ==
  Inertia : sm_lib/Body Elements/Inertia  InertiaType=Custom  Mass=0.28506911  MassUnits=kg  CenterOfMass=[0, 0, 0]  CenterOfMassUnits=m  MomentsOfInertia=[0.00040678, 0.00039958, 0.00059825]  MomentsOfInertiaUnits=kg*m^2  ProductsOfInertia=[-3.453e-05, -4e-08, 0]  ProductsOfInertiaUnits=kg*m^2  GraphicType=None  MarkerShape=Inertia  MarkerSize=20  GraphicVisPropType=SimpleVisualProperties  GraphicDiffuseColor=[0.5 0.5 0.5]  GraphicSpecularColor=[0.5 0.5 0.5 1.0]  GraphicAmbientColor=[0.15 0.15 0.15 1.0]  GraphicEmissiveColor=[0.0 0.0 0.0 1.0]  GraphicShininess=75  GraphicOpacity=1.0
  InertiaOriginTransform : sm_lib/Frames and Transforms/Rigid Transform  TranslationMethod=Cartesian  TranslationStandardOffset=0  TranslationLengthUnit=m  TranslationStandardAxis=+Z  TranslationCartesianOffset=[0, -0.03225261, -0.01842117]  TranslationROffset=0  TranslationROffsetUnits=m  TranslationZOffset=0  TranslationZOffsetUnits=m  TranslationThetaOffset=0  TranslationThetaOffsetUnits=deg  RotationMethod=RotationSequence  RotationAngleUnits=deg  RotationStandardAxis=+Z  RotationAngle=0.0  RotationArbitraryAxis=[0 0 1]  FollAlignAxisA=+X  BaseAlignAxisA=+Y  FollAlignAxisB=+Y  BaseAlignAxisB=+Z  RotationSequenceAxes=BaseAxes  RotationSequence=XYZ  RotationSequenceAngles=[0, 0, 0]  RotationSequenceAnglesUnits=rad  RotationMatrix=[1 0 0; 0 1 0; 0 0 1]
  ReferenceFrame : sm_lib/Frames and Transforms/Reference Frame
  shoulder_pitch_joint_AxisTransform : sm_lib/Frames and Transforms/Rigid Transform  TranslationMethod=Cartesian  TranslationStandardOffset=0  TranslationLengthUnit=m  TranslationStandardAxis=+Z  TranslationCartesianOffset=[0, 0, 0]  TranslationROffset=0  TranslationROffsetUnits=m  TranslationZOffset=0  TranslationZOffsetUnits=m  TranslationThetaOffset=0  TranslationThetaOffsetUnits=deg  RotationMethod=ArbitraryAxis  RotationAngleUnits=rad  RotationStandardAxis=+Z  RotationAngle=0  RotationArbitraryAxis=[1, 0, 0]  FollAlignAxisA=+X  BaseAlignAxisA=+Y  FollAlignAxisB=+Y  BaseAlignAxisB=+Z  RotationSequenceAxes=FollowerAxes  RotationSequence=XYX  RotationSequenceAngles=[0 0 0]  RotationSequenceAnglesUnits=deg  RotationMatrix=[1 0 0; 0 1 0; 0 0 1]
  shoulder_pitch_joint_OriginTransform : sm_lib/Frames and Transforms/Rigid Transform  TranslationMethod=Cartesian  TranslationStandardOffset=0  TranslationLengthUnit=m  TranslationStandardAxis=+Z  TranslationCartesianOffset=[0, -0.08500000000000001, 0]  TranslationROffset=0  TranslationROffsetUnits=m  TranslationZOffset=0  TranslationZOffsetUnits=m  TranslationThetaOffset=0  TranslationThetaOffsetUnits=deg  RotationMethod=RotationSequence  RotationAngleUnits=deg  RotationStandardAxis=+Z  RotationAngle=0.0  RotationArbitraryAxis=[0 0 1]  FollAlignAxisA=+X  BaseAlignAxisA=+Y  FollAlignAxisB=+Y  BaseAlignAxisB=+Z  RotationSequenceAxes=BaseAxes  RotationSequence=XYZ  RotationSequenceAngles=[-1.57, 0, 0]  RotationSequenceAnglesUnits=rad  RotationMatrix=[1 0 0; 0 1 0; 0 0 1]
  shoulder_roll_joint_AxisInvTransform : sm_lib/Frames and Transforms/Rigid Transform  TranslationMethod=Cartesian  TranslationStandardOffset=0  TranslationLengthUnit=m  TranslationStandardAxis=+Z  TranslationCartesianOffset=[0, 0, 0]  TranslationROffset=0  TranslationROffsetUnits=m  TranslationZOffset=0  TranslationZOffsetUnits=m  TranslationThetaOffset=0  TranslationThetaOffsetUnits=deg  RotationMethod=ArbitraryAxis  RotationAngleUnits=rad  RotationStandardAxis=+Z  RotationAngle=0  RotationArbitraryAxis=[1, 0, 0]  FollAlignAxisA=+X  BaseAlignAxisA=+Y  FollAlignAxisB=+Y  BaseAlignAxisB=+Z  RotationSequenceAxes=FollowerAxes  RotationSequence=XYX  RotationSequenceAngles=[0 0 0]  RotationSequenceAnglesUnits=deg  RotationMatrix=[1 0 0; 0 1 0; 0 0 1]
  F : PMIOPort  Side=Left
  F1 : PMIOPort  Port=2  Side=Right
  connections:
  Inertia/RConn1 -- InertiaOriginTransform/RConn1
  InertiaOriginTransform/LConn1 -- shoulder_pitch_joint_OriginTransform/LConn1 -- shoulder_roll_joint_AxisInvTransform/LConn1 -- ReferenceFrame/RConn1
  shoulder_pitch_joint_AxisTransform/RConn1 -- F1/RConn1
  shoulder_pitch_joint_AxisTransform/LConn1 -- shoulder_pitch_joint_OriginTransform/RConn1
  shoulder_roll_joint_AxisInvTransform/RConn1 -- F/RConn1

== system Comparision/DynamicCompansation/Robot/DynamicModel/dummy ==
  ReferenceFrame : sm_lib/Frames and Transforms/Reference Frame
  shoulder_roll_joint_AxisTransform : sm_lib/Frames and Transforms/Rigid Transform  TranslationMethod=Cartesian  TranslationStandardOffset=0  TranslationLengthUnit=m  TranslationStandardAxis=+Z  TranslationCartesianOffset=[0, 0, 0]  TranslationROffset=0  TranslationROffsetUnits=m  TranslationZOffset=0  TranslationZOffsetUnits=m  TranslationThetaOffset=0  TranslationThetaOffsetUnits=deg  RotationMethod=ArbitraryAxis  RotationAngleUnits=rad  RotationStandardAxis=+Z  RotationAngle=0  RotationArbitraryAxis=[1, 0, 0]  FollAlignAxisA=+X  BaseAlignAxisA=+Y  FollAlignAxisB=+Y  BaseAlignAxisB=+Z  RotationSequenceAxes=FollowerAxes  RotationSequence=XYX  RotationSequenceAngles=[0 0 0]  RotationSequenceAnglesUnits=deg  RotationMatrix=[1 0 0; 0 1 0; 0 0 1]
  shoulder_roll_joint_OriginTransform : sm_lib/Frames and Transforms/Rigid Transform  TranslationMethod=Cartesian  TranslationStandardOffset=0  TranslationLengthUnit=m  TranslationStandardAxis=+Z  TranslationCartesianOffset=[0, -0.1437625, 0.01166]  TranslationROffset=0  TranslationROffsetUnits=m  TranslationZOffset=0  TranslationZOffsetUnits=m  TranslationThetaOffset=0  TranslationThetaOffsetUnits=deg  RotationMethod=RotationSequence  RotationAngleUnits=deg  RotationStandardAxis=+Z  RotationAngle=0.0  RotationArbitraryAxis=[0 0 1]  FollAlignAxisA=+X  BaseAlignAxisA=+Y  FollAlignAxisB=+Y  BaseAlignAxisB=+Z  RotationSequenceAxes=BaseAxes  RotationSequence=XYZ  RotationSequenceAngles=[0, -1.57, 0]  RotationSequenceAnglesUnits=rad  RotationMatrix=[1 0 0; 0 1 0; 0 0 1]
  F : PMIOPort  Side=Left
  F1 : PMIOPort  Port=2  Side=Right
  connections:
  ReferenceFrame/RConn1 -- shoulder_roll_joint_OriginTransform/LConn1 -- F/RConn1
  shoulder_roll_joint_AxisTransform/RConn1 -- F1/RConn1
  shoulder_roll_joint_AxisTransform/LConn1 -- shoulder_roll_joint_OriginTransform/RConn1

== system Comparision/DynamicCompansation/Robot/DynamicModel/dummy2 ==
  ReferenceFrame : sm_lib/Frames and Transforms/Reference Frame
  F : PMIOPort  Side=Left
  connections:
  ReferenceFrame/RConn1 -- F/RConn1

== system Comparision/DynamicCompansation/Robot/DynamicModel/forearm_lower_link ==
  Inertia : sm_lib/Body Elements/Inertia  InertiaType=Custom  Mass=0.1177  MassUnits=kg  CenterOfMass=[0, 0, 0]  CenterOfMassUnits=m  MomentsOfInertia=[0.54274952, 1.03078569, 0.00010905]  MomentsOfInertiaUnits=kg*m^2  ProductsOfInertia=[0, 0, 0]  ProductsOfInertiaUnits=kg*m^2  GraphicType=None  MarkerShape=Inertia  MarkerSize=20  GraphicVisPropType=SimpleVisualProperties  GraphicDiffuseColor=[0.5 0.5 0.5]  GraphicSpecularColor=[0.5 0.5 0.5 1.0]  GraphicAmbientColor=[0.15 0.15 0.15 1.0]  GraphicEmissiveColor=[0.0 0.0 0.0 1.0]  GraphicShininess=75  GraphicOpacity=1.0
  InertiaOriginTransform : sm_lib/Frames and Transforms/Rigid Transform  TranslationMethod=Cartesian  TranslationStandardOffset=0  TranslationLengthUnit=m  TranslationStandardAxis=+Z  TranslationCartesianOffset=[0, -1.84e-06, -0.03625492]  TranslationROffset=0  TranslationROffsetUnits=m  TranslationZOffset=0  TranslationZOffsetUnits=m  TranslationThetaOffset=0  TranslationThetaOffsetUnits=deg  RotationMethod=RotationSequence  RotationAngleUnits=deg  RotationStandardAxis=+Z  RotationAngle=0.0  RotationArbitraryAxis=[0 0 1]  FollAlignAxisA=+X  BaseAlignAxisA=+Y  FollAlignAxisB=+Y  BaseAlignAxisB=+Z  RotationSequenceAxes=BaseAxes  RotationSequence=XYZ  RotationSequenceAngles=[0, 0, 0]  RotationSequenceAnglesUnits=rad  RotationMatrix=[1 0 0; 0 1 0; 0 0 1]
  ReferenceFrame : sm_lib/Frames and Transforms/Reference Frame
  elbow_yaw_joint_AxisInvTransform : sm_lib/Frames and Transforms/Rigid Transform  TranslationMethod=Cartesian  TranslationStandardOffset=0  TranslationLengthUnit=m  TranslationStandardAxis=+Z  TranslationCartesianOffset=[0, 0, 0]  TranslationROffset=0  TranslationROffsetUnits=m  TranslationZOffset=0  TranslationZOffsetUnits=m  TranslationThetaOffset=0  TranslationThetaOffsetUnits=deg  RotationMethod=ArbitraryAxis  RotationAngleUnits=rad  RotationStandardAxis=+Z  RotationAngle=0  RotationArbitraryAxis=[1, 0, 0]  FollAlignAxisA=+X  BaseAlignAxisA=+Y  FollAlignAxisB=+Y  BaseAlignAxisB=+Z  RotationSequenceAxes=FollowerAxes  RotationSequence=XYX  RotationSequenceAngles=[0 0 0]  RotationSequenceAnglesUnits=deg  RotationMatrix=[1 0 0; 0 1 0; 0 0 1]
  wrist_joint_OriginTransform : sm_lib/Frames and Transforms/Rigid Transform  TranslationMethod=Cartesian  TranslationStandardOffset=0  TranslationLengthUnit=m  TranslationStandardAxis=+Z  TranslationCartesianOffset=[0, 0, -0.05124]  TranslationROffset=0  TranslationROffsetUnits=m  TranslationZOffset=0  TranslationZOffsetUnits=m  TranslationThetaOffset=0  TranslationThetaOffsetUnits=deg  RotationMethod=RotationSequence  RotationAngleUnits=deg  RotationStandardAxis=+Z  RotationAngle=0.0  RotationArbitraryAxis=[0 0 1]  FollAlignAxisA=+X  BaseAlignAxisA=+Y  FollAlignAxisB=+Y  BaseAlignAxisB=+Z  RotationSequenceAxes=BaseAxes  RotationSequence=XYZ  RotationSequenceAngles=[1.5708, -1.5708, 0]  RotationSequenceAnglesUnits=rad  RotationMatrix=[1 0 0; 0 1 0; 0 0 1]
  F : PMIOPort  Side=Left
  F1 : PMIOPort  Port=2  Side=Right
  connections:
  Inertia/RConn1 -- InertiaOriginTransform/RConn1
  InertiaOriginTransform/LConn1 -- ReferenceFrame/RConn1 -- elbow_yaw_joint_AxisInvTransform/LConn1 -- wrist_joint_OriginTransform/LConn1
  elbow_yaw_joint_AxisInvTransform/RConn1 -- F/RConn1
  wrist_joint_OriginTransform/RConn1 -- F1/RConn1
